simulink model "task_3_scheme_CD"  (R2024a)
settings: Solver=FixedStepAuto  StartTime=0.0  StopTime=15.0  FixedStep=1e-4  RelTol=1e-3
settings Model: Creator=alexe  LastModifiedBy=alexe

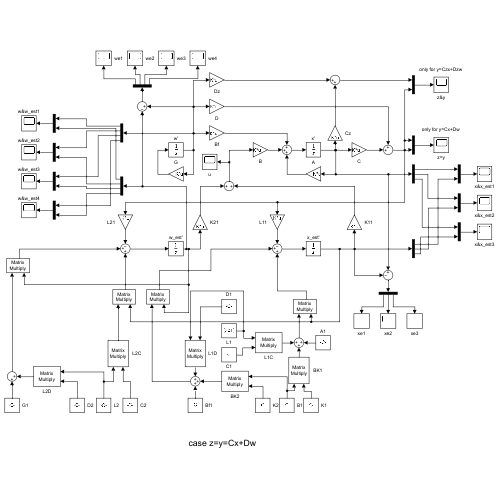
[thumbnail: Simulink's stored preview of the top-level diagram]
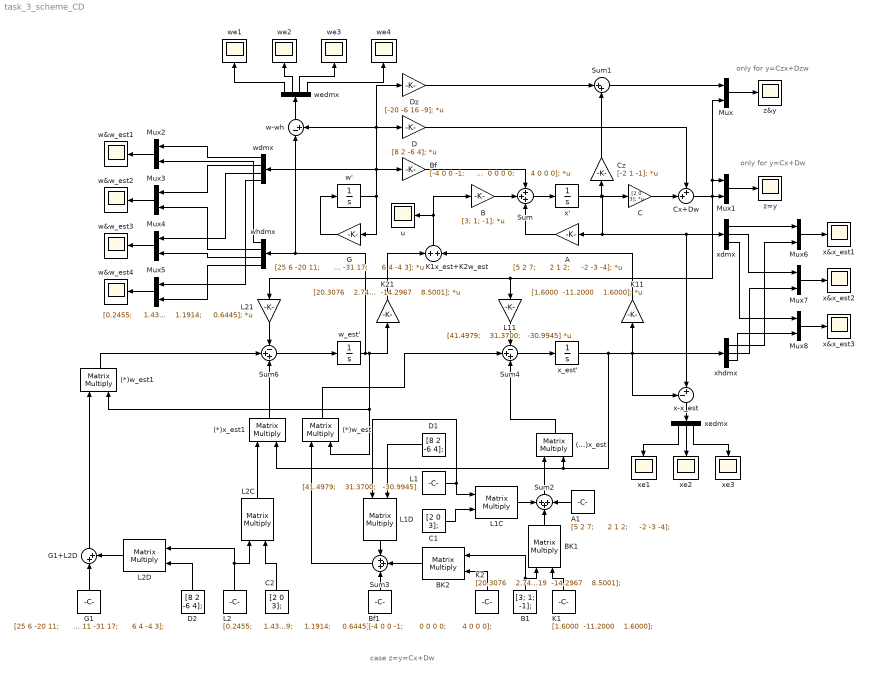
== system task_3_scheme_CD ==
  note: only for y=Czx+Dzw
  note: case z=y=Cx+Dw
  note: only for y=Cx+Dw
  " BK1" : Product  Multiplication=Matrix(*)
  " L2C" : Product  Multiplication=Matrix(*)
  (*)w_est : Product  Multiplication=Matrix(*)
  (*)w_est1 : Product  Multiplication=Matrix(*)
  (*)x_est1 : Product  Multiplication=Matrix(*)
  (...)x_est : Product  Multiplication=Matrix(*)
  A : Gain  Gain=|  Multiplication=Matrix(K*u)
      | [5 2 7;
      |      2 1 2;
      |     -2 -3 -4];
  A1 : Constant  Value=|  VectorParams1D=off
      | [5 2 7;
      |      2 1 2;
      |     -2 -3 -4];
  B : Gain  Gain=[3; 1; -1];  Multiplication=Matrix(K*u)
  B1 : Constant  Value=[3; 1; -1];  VectorParams1D=off
  BK2 : Product  Multiplication=Matrix(*)
  Bf : Gain  Gain=|  Multiplication=Matrix(K*u)
      | [-4 0 0 -1;
      |       0 0 0 0;
      |       4 0 0 0];
  Bf1 : Constant  Value=|  VectorParams1D=off
      | [-4 0 0 -1;
      |       0 0 0 0;
      |       4 0 0 0];
  C : Gain  Gain=[2 0 3];  Multiplication=Matrix(K*u)
  C1 : Constant  Value=[2 0 3];  VectorParams1D=off
  C2 : Constant  Value=[2 0 3];  VectorParams1D=off
  Cx+Dw : Sum  Inputs=++|
  Cz : Gain  Gain=[-2 1 -1];  Multiplication=Matrix(K*u)
  D : Gain  Gain=[8 2 -6 4];  Multiplication=Matrix(K*u)
  D1 : Constant  Value=[8 2 -6 4];  VectorParams1D=off
  D2 : Constant  Value=[8 2 -6 4];  VectorParams1D=off
  Dz : Gain  Gain=[-20 -6 16 -9];  Multiplication=Matrix(K*u)
  G : Gain  Gain=|  Multiplication=Matrix(K*u)
      | [25 6 -20 11;
      |      14 3 -10 4;
      |      40 11 -31 17;
      |      6 4 -4 3];
  G1 : Constant  Value=|  VectorParams1D=off
      | [25 6 -20 11;
      |      14 3 -10 4;
      |      40 11 -31 17;
      |      6 4 -4 3];
  G1+L2D : Sum  Inputs=|++
  K1 : Constant  Value="[1.6000  -11.2000    1.6000];"  VectorParams1D=off
  K11 : Gain  Gain="[1.6000  -11.2000    1.6000];"  Multiplication=Matrix(K*u)
  K1x_est+K2w_est : Sum
  K2 : Constant  Value="[20.3076    2.7419  -14.2967    8.5001];"  VectorParams1D=off
  K21 : Gain  Gain="[20.3076    2.7419  -14.2967    8.5001];"  Multiplication=Matrix(K*u)
  L1 : Constant  Value=|  VectorParams1D=off
      | [41.4979;
      |    31.3700;
      |   -30.9945]
  L11 : Gain  Gain=|  Multiplication=Matrix(K*u)
      | [41.4979;
      |    31.3700;
      |   -30.9945]
  L1C : Product  Multiplication=Matrix(*)
  L1D : Product  Multiplication=Matrix(*)
  L2 : Constant  Value=|  VectorParams1D=off
      | [0.2455;
      |     1.4359;
      |     1.1914;
      |     0.6445];
  L21 : Gain  Gain=|  Multiplication=Matrix(K*u)
      | [0.2455;
      |     1.4359;
      |     1.1914;
      |     0.6445];
  L2D : Product  Multiplication=Matrix(*)
  Mux{,1..8} (9 alike) : Mux  Inputs=2
  Sum : Sum  Inputs=+++
  Sum1 : Sum  Inputs=|++
  Sum2 : Sum  Inputs=+++
  Sum3 : Sum  Inputs=+++
  Sum4 : Sum  Inputs=-++
  Sum6 : Sum  Inputs=-++
  u : Scope
  w&w_est{1..4} (4 alike) : Scope
  w' : Integrator  InitialCondition=[1;1;1;1]
  w-wh : Sum  Inputs=|-+
  w_est' : Integrator  InitialCondition=[0;0;0;0]
  wdmx : Demux
  we{1..4} (4 alike) : Scope
  wedmx : Demux
  whdmx : Demux
  x&x_est1 : Scope
  x&x_est2 : Scope
  x&x_est3 : Scope
  x' : Integrator  InitialCondition=[0;0;0]
  x-x_est : Sum  Inputs=-+|
  x_est' : Integrator  InitialCondition=[0;0;0]
  xdmx : Demux  Outputs=3
  xe1 : Scope
  xe2 : Scope
  xe3 : Scope
  xedmx : Demux  Outputs=3
  xhdmx : Demux  Outputs=3
  z&y : Scope
  z=y : Scope
  wires:
  x'/1 -> x-x_est/2, xdmx/1, A/1, C/1, Cz/1
  Sum/1 -> x'/1
  w'/1 -> wdmx/1, w-wh/2, D/1, Dz/1, Bf/1, G/1
  G/1 -> w'/1
  A/1 -> Sum/3
  B/1 -> Sum/2
  Bf/1 -> Sum/1
  D/1 -> Cx+Dw/1
  C/1 -> Cx+Dw/2
  x_est'/1 -> x-x_est/1, xhdmx/1, K11/1, (*)x_est1/2, (...)x_est/2
  " BK1"/1 -> Sum2/2
  K1/1 -> " BK1"/2
  L1/1 -> L1D/1, L1C/1
  C1/1 -> L1C/2
  L1C/1 -> Sum2/1
  A1/1 -> Sum2/3
  Sum2/1 -> (...)x_est/1
  B1/1 -> " BK1"/1, BK2/1
  K2/1 -> BK2/2
  D1/1 -> L1D/2
  Bf1/1 -> Sum3/3
  L1D/1 -> Sum3/1
  BK2/1 -> Sum3/2
  Sum3/1 -> (*)w_est/1
  w_est'/1 -> K21/1, (*)w_est/2, (*)w_est1/2, w-wh/1, whdmx/1
  L11/1 -> Sum4/1
  Cx+Dw/1 -> Mux1/2, Mux1/1, Mux/2, L21/1, L11/1
  (...)x_est/1 -> Sum4/3
  (*)w_est/1 -> Sum4/2
  Sum4/1 -> x_est'/1
  L2/1 -> L2D/1, " L2C"/1
  C2/1 -> " L2C"/2
  " L2C"/1 -> (*)x_est1/1
  D2/1 -> L2D/2
  L2D/1 -> G1+L2D/2
  G1/1 -> G1+L2D/1
  G1+L2D/1 -> (*)w_est1/1
  L21/1 -> Sum6/1
  Sum6/1 -> w_est'/1
  (*)x_est1/1 -> Sum6/3
  (*)w_est1/1 -> Sum6/2
  K21/1 -> K1x_est+K2w_est/1
  K11/1 -> K1x_est+K2w_est/2
  K1x_est+K2w_est/1 -> u/1, B/1
  Cz/1 -> Sum1/2
  Dz/1 -> Sum1/1
  Mux/1 -> z&y/1
  Sum1/1 -> Mux/1
  Mux1/1 -> z=y/1
  Mux5/1 -> w&w_est4/1
  Mux4/1 -> w&w_est3/1
  Mux3/1 -> w&w_est2/1
  Mux2/1 -> w&w_est1/1
  wdmx/1 -> Mux2/1
  whdmx/1 -> Mux2/2
  wdmx/2 -> Mux3/1
  whdmx/2 -> Mux3/2
  wdmx/3 -> Mux4/1
  whdmx/3 -> Mux4/2
  wdmx/4 -> Mux5/1
  whdmx/4 -> Mux5/2
  Mux8/1 -> x&x_est3/1
  Mux7/1 -> x&x_est2/1
  Mux6/1 -> x&x_est1/1
  xdmx/1 -> Mux6/1
  xhdmx/1 -> Mux6/2
  xdmx/2 -> Mux7/1
  xhdmx/2 -> Mux7/2
  xdmx/3 -> Mux8/1
  xhdmx/3 -> Mux8/2
  w-wh/1 -> wedmx/1
  wedmx/1 -> we1/1
  wedmx/2 -> we2/1
  wedmx/3 -> we3/1
  wedmx/4 -> we4/1
  x-x_est/1 -> xedmx/1
  xedmx/1 -> xe1/1
  xedmx/2 -> xe2/1
  xedmx/3 -> xe3/1
